simulink model "division2_repro"  (R2025b)
settings: Solver=ode4  StartTime=0.0  StopTime=40  FixedStep=dt  RelTol=1e-3
undefined symbols (not defined in the file): a0, a1, a2, a3, a4, a5, a6, a7, AgN, AgP, CNrt, CPrt, dt, EQ_intensity, EQ_sw, feedthrough_matrix_cb, feedthrough_matrix_guyan, feedthrough_matrix_original, G_1, G_2, G_3, Gss, Gss_1, KNbar_inv, KPbar_inv, KPrt, KRrt, lN, locate, locate3, lP, Mf, MNrt, MPrt, MRrt, output_matrix_cb, output_matrix_guyan, output_matrix_original, RNbar, RPbar, T, T_cb
libraries: simulink x1, sldrtlib x1
settings Model: Creator=icu327  LastModifiedBy=lenovo
settings DataIOCC: SaveFormat=Array  ReturnWorkspaceOutputs=off
settings DebuggingCC: UnconnectedInputMsg=warning  UnconnectedOutputMsg=warning  UnconnectedLineMsg=warning  ArithmeticOperatorsInVariantConditions=warning
settings HardwareCC: ProdBitPerLong=64.0  ProdHWDeviceType=Intel->x86-64 (Linux 64)
settings ModelReferenceCC: EnableRefExpFcnMdlSchedulingChecks=on
settings SFSimCC: CustomCodeUndefinedFunction=UseInterfaceOnly
settings RTWCC: SystemTargetFile=sldrt.tlc  TemplateMakefile=sldrt.tmf  RTWCompilerOptimization=on  GPUComputeCapability=3.5  Description=Simulink Desktop Real-Time
settings CodeAppCC: MaxIdLength=95.0  StateflowObjectComments=on
settings SimulinkDesktopRealTimeCC: ExtModeTransport=0.0  ExtModeStaticAllocSize=1000000.0  TargetLibSuffix=_sldrt.a  TargetPreCompLibLocation=D:\Downlad\Matlab\toolbox\sldrt\lib\win64  MultiwordLength=2048.0  DynamicStringBufferSize=256.0  ParMdlRefBuildCompliant=on  PreserveMATLABNamespacesInGeneratedCode=on  SubcomponentCodeInterfacePackaging=Reusable function

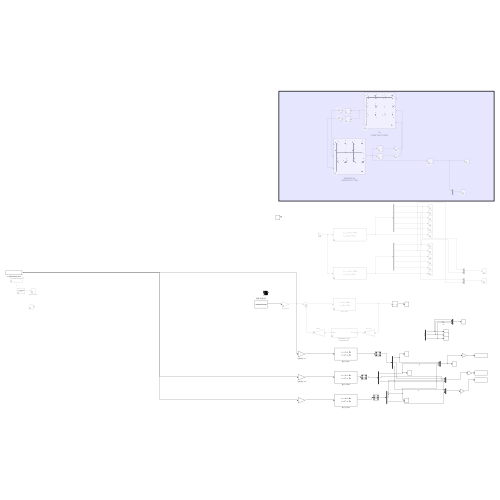
[thumbnail: Simulink's stored preview of the top-level diagram]
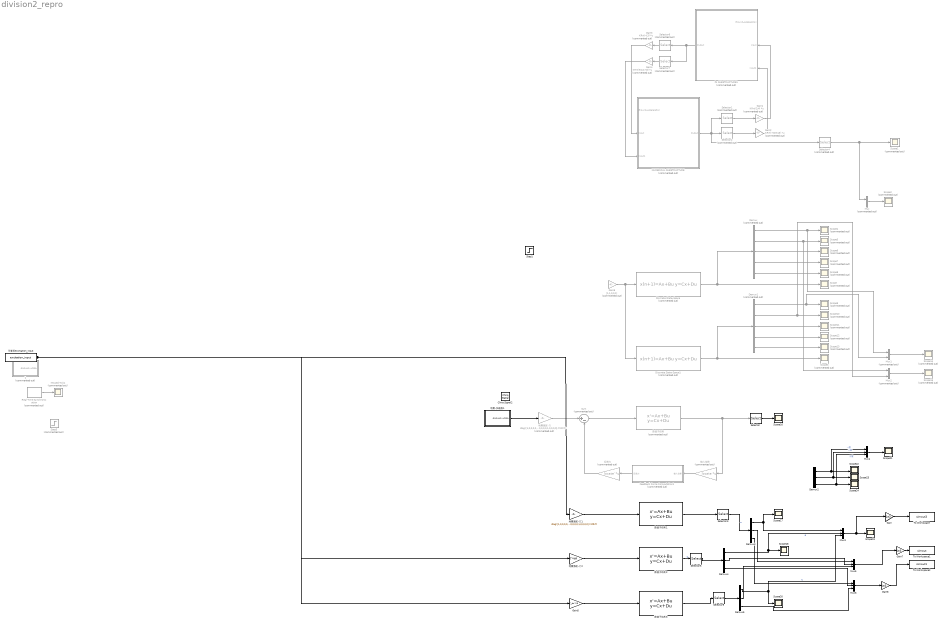
== system division2_repro ==
  " 1" : Subsystem  Commented=on
  " NUMERICAL SUBSTRUCTURE" : Subsystem  Commented=on
      mask Display: image('$imagefile'); % Use "Edit Image" on toolstrip to change.
  " Ps SUBSTRUCTURE1" : Subsystem  Commented=on
      mask Display: image('$imagefile'); % Use "Edit Image" on toolstrip to change.
  " 地震-加速度1" : Subsystem
  Chirp Signal2 : simulink/Sources/Chirp Signal  f1=0.1  T=40  f2=10
  Demux : Demux  Commented=on  Outputs=5
  Demux1 : Demux  Commented=on  Outputs=5
  Demux{2..5} (4 alike) : Demux  Outputs=3
  Discrete State-Space : DiscreteStateSpace  Commented=on  A=Gss.A  B=Gss.B  C=Gss.C  D=Gss.D  SampleTime=-1
  Discrete State-Space1 : DiscreteStateSpace  Commented=on  A=Gss_1.A  B=Gss_1.B  C=Gss_1.C  D=Gss_1.D  SampleTime=-1
  Feedback Force Computation1 : Subsystem  Commented=on
  Gain : Gain  Gain=1e3
  Gain1 : Gain  Commented=on  Gain=KRrt(3,4)  Multiplication=Matrix(K*u) (u vector)
  Gain2 : Gain  Commented=on  Gain=KRrt(7:8,9:13)  Multiplication=Matrix(K*u) (u vector)
  Gain3 : Gain  Commented=on  Gain=KRrt(4,3)  Multiplication=Matrix(K*u) (u vector)
  Gain4 : Gain  Commented=on  Gain=KRrt(9:13,7:8)  Multiplication=Matrix(K*u) (u vector)
  Gain5 : Gain  Gain=T_cb'*Mf
  Gain6 : Gain  Commented=on  Gain=[1,1,0,0,1]
  Gain7 : Gain  Gain=1e3
  Gain8 : Gain  Gain=1e3
  Missed Ticks : Scope  Commented=on
      settings: ActiveDisplayYMinimum=-21.375  ActiveDisplayYMaximum=192.375
  Mux : Mux  Commented=on  Inputs=2
  Mux1 : Mux  Commented=on  Inputs=2
  Mux2 : Mux  Commented=on  Inputs=2
  Mux{3..6} (4 alike) : Mux  Inputs=3
  Real-Time Synchronization : sldrtlib/Real-Time Synchronization  Commented=on  SampleTime=dt  MaxMissedTicks=10000  ShowMissedTicks=on  YieldWhenWaiting=off
  Scope{,1..15} (16 alike) : Scope  Commented=on
      Scope settings: ActiveDisplayYMinimum=-8E-7  ActiveDisplayYMaximum=7E-7
      Scope1 settings: ActiveDisplayYMinimum=-448565.92172  ActiveDisplayYMaximum=49840.65797
      Scope10 settings: ActiveDisplayYMinimum=-3.7E-6  ActiveDisplayYMaximum=3.7E-6
      Scope11 settings: ActiveDisplayYMinimum=-6E-6  ActiveDisplayYMaximum=6E-6  DataLoggingVariableName=ScopeData2
      Scope12 settings: ActiveDisplayYMinimum=-7E-6  ActiveDisplayYMaximum=7E-6  DataLoggingVariableName=ScopeData3
      Scope13 settings: ActiveDisplayYMinimum=-7E-7  ActiveDisplayYMaximum=7E-7  DataLoggingVariableName=ScopeData4
      Scope14 settings: ActiveDisplayYMinimum=-6E-7  ActiveDisplayYMaximum=7E-7  DataLoggingVariableName=ScopeData7
      Scope15 settings: ActiveDisplayYMinimum=-1.6E-6  ActiveDisplayYMaximum=1.7E-6
      Scope2 settings: ActiveDisplayYMinimum=-448565.92172  ActiveDisplayYMaximum=49840.65797  DataLoggingVariableName=ScopeData2
      Scope3 settings: ActiveDisplayYMinimum=-2.5E-6  ActiveDisplayYMaximum=2.5E-6  DataLoggingVariableName=ScopeData5
      Scope4 settings: ActiveDisplayYMinimum=-2.5E-8  ActiveDisplayYMaximum=3.7E-8  DataLoggingVariableName=ScopeData3
      Scope5 settings: ActiveDisplayYMinimum=-3.7E-6  ActiveDisplayYMaximum=3.7E-6  DataLoggingVariableName=ScopeData4
      Scope6 settings: ActiveDisplayYMinimum=-6E-6  ActiveDisplayYMaximum=6E-6  DataLoggingVariableName=ScopeData5
      Scope7 settings: ActiveDisplayYMinimum=-7E-6  ActiveDisplayYMaximum=7E-6  DataLoggingVariableName=ScopeData6
      Scope8 settings: ActiveDisplayYMinimum=-7E-7  ActiveDisplayYMaximum=7E-7  DataLoggingVariableName=ScopeData7
      Scope9 settings: ActiveDisplayYMinimum=-2.5E-8  ActiveDisplayYMaximum=3.7E-8  DataLoggingVariableName=ScopeData6
  Scope{16..24} (9 alike) : Scope
      Scope16 settings: ActiveDisplayYMinimum=-4.1813024288037124E+278  ActiveDisplayYMaximum=3.7631721859233419E+279
      Scope17 settings: ActiveDisplayYMinimum=-0.00351  ActiveDisplayYMaximum=0.00404
      Scope18 settings: ActiveDisplayYMinimum=-0.00375  ActiveDisplayYMaximum=0.00378  DataLoggingVariableName=ScopeData2
      Scope19 settings: ActiveDisplayYMinimum=-0.01112  ActiveDisplayYMaximum=0.00785  DataLoggingVariableName=ScopeData3
      Scope20 settings: ActiveDisplayYMinimum=-0.00351  ActiveDisplayYMaximum=0.00404  DataLoggingVariableName=ScopeData4
      Scope21 settings: ActiveDisplayYMinimum=-0.01512  ActiveDisplayYMaximum=0.0154
      Scope22 settings: ActiveDisplayYMinimum=-0.00351  ActiveDisplayYMaximum=0.00405  DataLoggingVariableName=ScopeData2
      Scope23 settings: ActiveDisplayYMinimum=-0.00973  ActiveDisplayYMaximum=0.01044  DataLoggingVariableName=ScopeData3
      Scope24 settings: ActiveDisplayYMinimum=-0.01512  ActiveDisplayYMaximum=0.0154  DataLoggingVariableName=ScopeData4
  Selector : Selector  InputPortWidth=15  IndexOptions=Index vector (dialog)  Indices=[1]  OutputSizes=1
  Selector1 : Selector  Commented=on  InputPortWidth=11  IndexOptions=Index vector (dialog)  Indices=[2]  OutputSizes=1
  Selector2 : Selector  Commented=on  InputPortWidth=11  IndexOptions=Index vector (dialog)  Indices=[5 6 7 8 9]  OutputSizes=1
  Selector3 : Selector  InputPortWidth=3  IndexOptions=Index vector (dialog)  Indices=[1 2 3]  OutputSizes=1
  Selector4 : Selector  Commented=on  InputPortWidth=11  IndexOptions=Index vector (dialog)  Indices=[1]  OutputSizes=1
  Selector5 : Selector  InputPortWidth=3  IndexOptions=Index vector (dialog)  Indices=[1 2 3]  OutputSizes=1
  Selector6 : Selector  Commented=on  InputPortWidth=6  IndexOptions=Index vector (dialog)  Indices=[3]  OutputSizes=1
  Selector7 : Selector  Commented=on  InputPortWidth=6  IndexOptions=Index vector (dialog)  Indices=[5 6]  OutputSizes=1
  Selector9 : Selector  InputPortWidth=3  IndexOptions=Index vector (dialog)  Indices=[1 2 3]  OutputSizes=1
  Step1 : Step  SampleTime=0
  Step5 : Step  Commented=on  SampleTime=0
  Sum : Sum  Commented=on  Inputs=|+-
  To Workspace : ToWorkspace  VariableName=simout3  SaveFormat=Timeseries  SampleTime=-1
  To Workspace1 : ToWorkspace  VariableName=simout  SaveFormat=Timeseries  SampleTime=-1
  To Workspace2 : ToWorkspace  VariableName=simout1  SaveFormat=Timeseries  SampleTime=-1
  反馈力 : Gain  Commented=on  Gain=locate'  Multiplication=Matrix(K*u) (u vector)
  可复现excitation_input : FromWorkspace  VariableName=excitation_input  OutputAfterFinalValue=Holding final value
  地震激励-力 : Gain  Commented=on  Gain=diag([1,0,0,0,0,1,0,0,0,0,1,0,0,0,0].*MRrt)
  地震激励-力1 : Gain  Gain=diag([1,0,0,0,0,1,0,0,0,0,1,0,0,0,0].*MRrt)
  地震激励-力2 : Gain  Gain=T'*Mf
  数值子结构 : StateSpace  Commented=on  InitialCondition=0
  数值子结构1 : StateSpace  A=G_1.A  B=G_1.B  C=output_matrix_original  D=feedthrough_matrix_original  InitialCondition=0
  数值子结构2 : StateSpace  A=G_2.A  B=G_2.B  C=output_matrix_guyan  D=feedthrough_matrix_guyan  InitialCondition=0
  数值子结构3 : StateSpace  A=G_3.A  B=G_3.B  C=output_matrix_cb  D=feedthrough_matrix_cb  InitialCondition=0
  输入位移 : Gain  Commented=on  Gain=locate  Multiplication=Matrix(K*u) (u vector)
  wires:
  Real-Time Synchronization/1 -> Missed Ticks/1
  Mux/1 -> Scope2/1
  " Ps SUBSTRUCTURE1"/1(Output) -> Selector7/1, Selector6/1
  Selector4/1 -> Scope1/1, Mux/1
  Selector2/1 -> Gain2/1
  Selector1/1 -> Gain1/1
  Gain1/1 -> " Ps SUBSTRUCTURE1"/2(Input)
  Gain2/1 -> " Ps SUBSTRUCTURE1"/3(Input1)
  Selector6/1 -> Gain3/1
  Gain3/1 -> " NUMERICAL SUBSTRUCTURE"/2(Input)
  Selector7/1 -> Gain4/1
  Gain4/1 -> " NUMERICAL SUBSTRUCTURE"/3(Input1)
  " NUMERICAL SUBSTRUCTURE"/1(Output) -> Selector4/1, Selector1/1, Selector2/1
  Discrete State-Space/1 -> Demux/1, Scope/1
  Demux/1 -> Mux1/1, Scope4/1
  Demux/2 -> Mux2/1, Scope5/1
  Demux/4 -> Scope7/1
  Demux/5 -> Scope8/1
  Demux1/5 -> Scope13/1
  Demux1/4 -> Scope12/1
  Demux1/1 -> Mux1/2, Scope9/1
  Discrete State-Space1/1 -> Demux1/1, Scope3/1
  Gain6/1 -> Discrete State-Space1/1, Discrete State-Space/1
  Demux1/3 -> Scope11/1
  Mux1/1 -> Scope14/1
  Mux2/1 -> Scope15/1
  Demux1/2 -> Mux2/2, Scope10/1
  Demux/3 -> Scope6/1
  Selector/1 -> Scope16/1
  数值子结构/1 -> 输入位移/1, Selector/1
  Feedback Force Computation1/1(反馈力) -> 反馈力/1
  输入位移/1 -> Feedback Force Computation1/1(输入位移)
  地震激励-力/1 -> Sum/1
  Sum/1 -> 数值子结构/1
  反馈力/1 -> Sum/2
  数值子结构1/1 -> Selector3/1
  地震激励-力1/1 -> 数值子结构1/1
  地震激励-力2/1 -> 数值子结构2/1
  Demux4/1 -> Scope18/1, Mux3/2  "g"
  Mux3/1 -> Gain/1, Scope19/1
  " 地震-加速度1"/1(GROUND ACCEL) -> 地震激励-力/1
  数值子结构3/1 -> Selector9/1
  Demux5/1 -> Mux3/3, Scope20/1  "C"
  Gain5/1 -> 数值子结构3/1
  Demux2/1 -> Mux4/1, Scope22/1  "一层"
  Demux2/2 -> Mux4/2, Scope23/1  "二层"
  Demux2/3 -> Mux4/3, Scope24/1  "三层"
  Mux4/1 -> Scope21/1
  Selector3/1 -> Demux3/1  "o"
  Demux3/1 -> Mux3/1, Scope17/1
  数值子结构2/1 -> Selector5/1  "g"
  Selector9/1 -> Demux5/1
  Demux3/2 -> Mux5/1
  Demux4/2 -> Mux5/2
  Demux5/2 -> Mux5/3
  Demux3/3 -> Mux6/1
  Mux5/1 -> Gain7/1
  Mux6/1 -> Gain8/1
  Gain/1 -> To Workspace/1
  Gain7/1 -> To Workspace1/1
  Gain8/1 -> To Workspace2/1
  Selector5/1 -> Demux4/1
  可复现excitation_input/1 -> 地震激励-力1/1, 地震激励-力2/1, Gain5/1
  Demux4/3 -> Mux6/2
  Demux5/3 -> Mux6/3

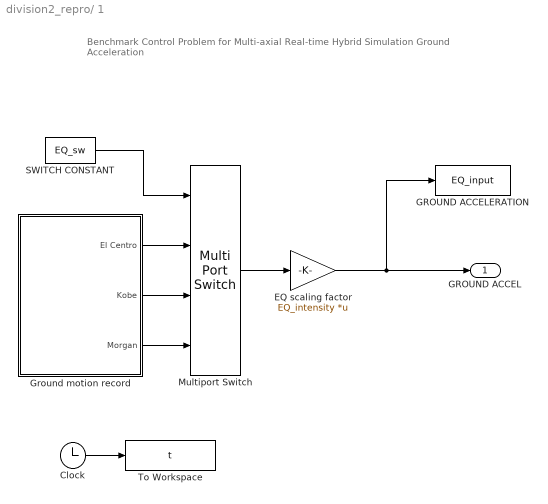
== system division2_repro/ 1 ==
  note: Benchmark Control Problem for
      | Multi-axial Real-time Hybrid Simulation
      | Ground Acceleration
  Clock : Clock
  EQ scaling factor : Gain  Gain=EQ_intensity  Multiplication=Matrix(K*u)
  GROUND ACCELERATION : ToWorkspace  VariableName=EQ_input  SampleTime=-1
      settings: Save2DSignal=2-D array (concatenate along first dimension)
  Ground motion record : Subsystem
  Multiport Switch : MultiPortSwitch  SaturateOnIntegerOverflow=off  InputSameDT=off
  SWITCH CONSTANT : Constant  Value=EQ_sw
  To Workspace : ToWorkspace  VariableName=t  SampleTime=dt
  GROUND ACCEL : Outport  VectorParamsAs1DForOutWhenUnconnected=off
  wires:
  Multiport Switch/1 -> EQ scaling factor/1
  EQ scaling factor/1 -> GROUND ACCELERATION/1, GROUND ACCEL/1
  Ground motion record/1(El Centro) -> Multiport Switch/2
  Ground motion record/2(Kobe) -> Multiport Switch/3
  Ground motion record/3(Morgan) -> Multiport Switch/4
  SWITCH CONSTANT/1 -> Multiport Switch/1
  Clock/1 -> To Workspace/1

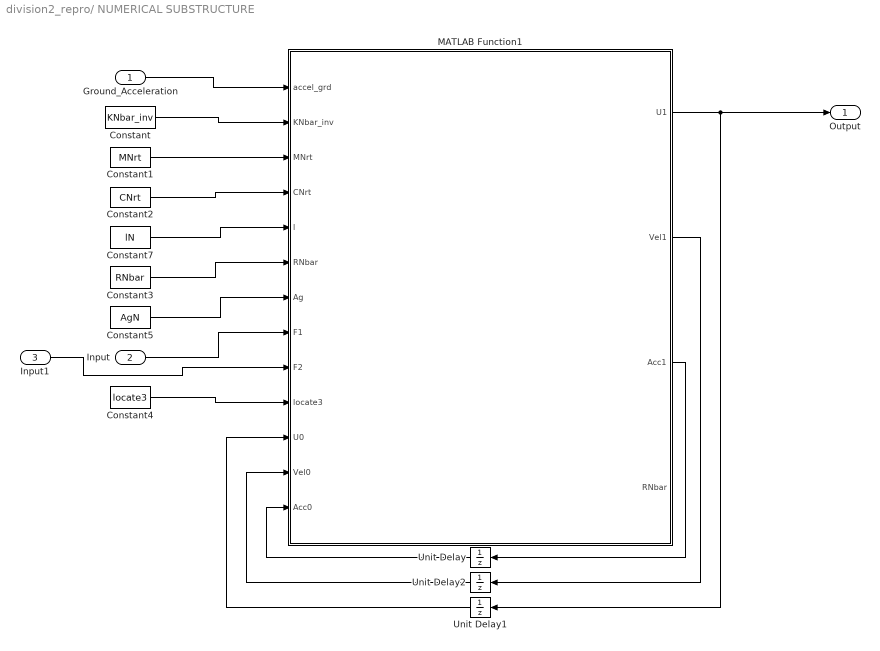
== system division2_repro/ NUMERICAL SUBSTRUCTURE ==
  Ground_Acceleration : Inport
  Input : Inport  Port=2
  Input1 : Inport  Port=3
  Constant : Constant  Value=KNbar_inv  VectorParams1D=off
  Constant1 : Constant  Value=MNrt  VectorParams1D=off
  Constant2 : Constant  Value=CNrt  VectorParams1D=off
  Constant3 : Constant  Value=RNbar  VectorParams1D=off
  Constant4 : Constant  Value=locate3  VectorParams1D=off
  Constant5 : Constant  Value=AgN  VectorParams1D=off
  Constant7 : Constant  Value=lN  VectorParams1D=off
  MATLAB Function1 : MATLAB Function  TreatAsAtomicUnit=on
  Unit Delay : UnitDelay  SampleTime=-1  HasFrameUpgradeWarning=on
  Unit Delay1 : UnitDelay  SampleTime=-1  HasFrameUpgradeWarning=on
  Unit Delay2 : UnitDelay  SampleTime=-1  HasFrameUpgradeWarning=on
  Output : Outport
  wires:
  Ground_Acceleration/1 -> MATLAB Function1/1(accel_grd)
  Constant/1 -> MATLAB Function1/2(KNbar_inv)
  Constant1/1 -> MATLAB Function1/3(MNrt)
  Constant2/1 -> MATLAB Function1/4(CNrt)
  Constant7/1 -> MATLAB Function1/5(l)
  Unit Delay2/1 -> MATLAB Function1/12(Vel0)
  Unit Delay/1 -> MATLAB Function1/13(Acc0)
  MATLAB Function1/2(Vel1) -> Unit Delay2/1
  MATLAB Function1/3(Acc1) -> Unit Delay/1
  Constant5/1 -> MATLAB Function1/7(Ag)
  Unit Delay1/1 -> MATLAB Function1/11(U0)
  Constant3/1 -> MATLAB Function1/6("RNbar ")
  Input/1 -> MATLAB Function1/8(F1)
  MATLAB Function1/1(U1) -> Output/1, Unit Delay1/1
  Constant4/1 -> MATLAB Function1/10(locate3)
  Input1/1 -> MATLAB Function1/9(F2)

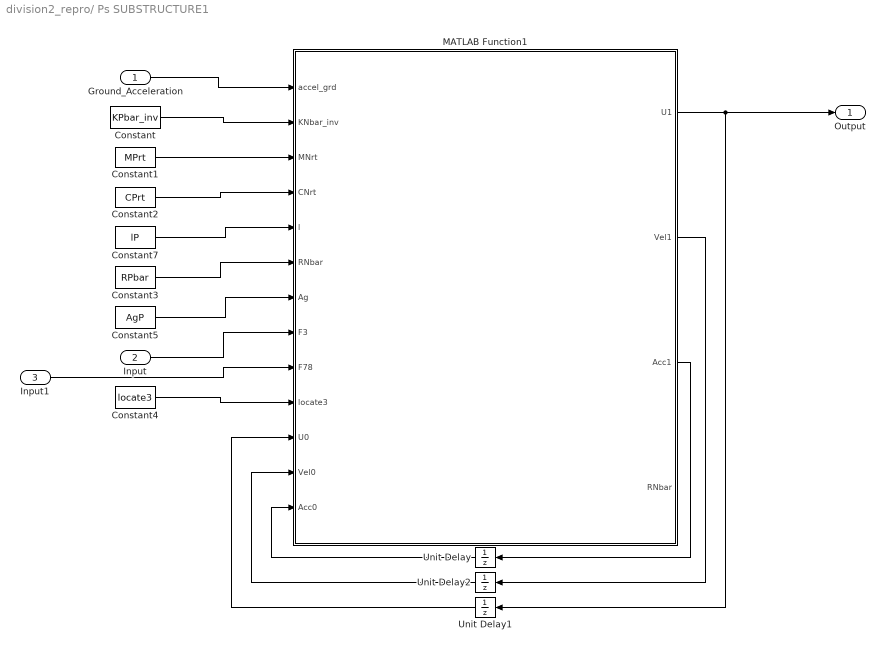
== system division2_repro/ Ps SUBSTRUCTURE1 ==
  Ground_Acceleration : Inport
  Input : Inport  Port=2
  Input1 : Inport  Port=3
  Constant : Constant  Value=KPbar_inv  VectorParams1D=off
  Constant1 : Constant  Value=MPrt  VectorParams1D=off
  Constant2 : Constant  Value=CPrt  VectorParams1D=off
  Constant3 : Constant  Value=RPbar  VectorParams1D=off
  Constant4 : Constant  Value=locate3  VectorParams1D=off
  Constant5 : Constant  Value=AgP  VectorParams1D=off
  Constant7 : Constant  Value=lP  VectorParams1D=off
  MATLAB Function1 : MATLAB Function  TreatAsAtomicUnit=on
  Unit Delay : UnitDelay  SampleTime=-1  HasFrameUpgradeWarning=on
  Unit Delay1 : UnitDelay  SampleTime=-1  HasFrameUpgradeWarning=on
  Unit Delay2 : UnitDelay  SampleTime=-1  HasFrameUpgradeWarning=on
  Output : Outport
  wires:
  Ground_Acceleration/1 -> MATLAB Function1/1(accel_grd)
  Constant/1 -> MATLAB Function1/2(KNbar_inv)
  Constant1/1 -> MATLAB Function1/3(MNrt)
  Constant2/1 -> MATLAB Function1/4(CNrt)
  Constant7/1 -> MATLAB Function1/5(l)
  Unit Delay2/1 -> MATLAB Function1/12(Vel0)
  Unit Delay/1 -> MATLAB Function1/13(Acc0)
  MATLAB Function1/2(Vel1) -> Unit Delay2/1
  MATLAB Function1/3(Acc1) -> Unit Delay/1
  Constant5/1 -> MATLAB Function1/7(Ag)
  Unit Delay1/1 -> MATLAB Function1/11(U0)
  Constant3/1 -> MATLAB Function1/6("RNbar ")
  Input/1 -> MATLAB Function1/8(F3)
  MATLAB Function1/1(U1) -> Output/1, Unit Delay1/1
  Constant4/1 -> MATLAB Function1/10(locate3)
  Input1/1 -> MATLAB Function1/9(F78)

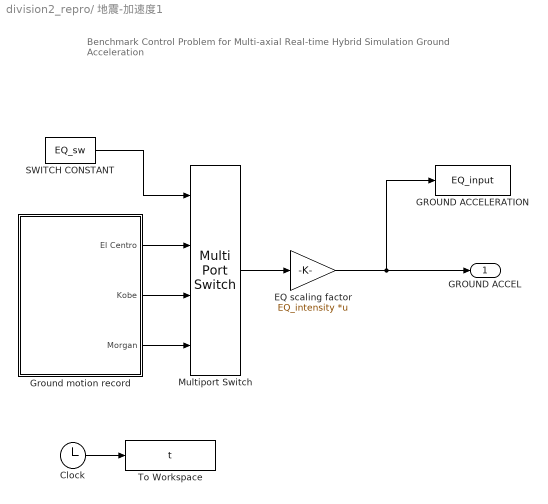
== system division2_repro/ 地震-加速度1 ==
  note: Benchmark Control Problem for
      | Multi-axial Real-time Hybrid Simulation
      | Ground Acceleration
  Clock : Clock
  EQ scaling factor : Gain  Gain=EQ_intensity  Multiplication=Matrix(K*u)
  GROUND ACCELERATION : ToWorkspace  VariableName=EQ_input  SampleTime=-1
      settings: Save2DSignal=2-D array (concatenate along first dimension)
  Ground motion record : Subsystem
  Multiport Switch : MultiPortSwitch  SaturateOnIntegerOverflow=off  InputSameDT=off
  SWITCH CONSTANT : Constant  Value=EQ_sw
  To Workspace : ToWorkspace  VariableName=t  SampleTime=dt
  GROUND ACCEL : Outport  VectorParamsAs1DForOutWhenUnconnected=off
  wires:
  Multiport Switch/1 -> EQ scaling factor/1
  EQ scaling factor/1 -> GROUND ACCELERATION/1, GROUND ACCEL/1
  Ground motion record/1(El Centro) -> Multiport Switch/2
  Ground motion record/2(Kobe) -> Multiport Switch/3
  Ground motion record/3(Morgan) -> Multiport Switch/4
  SWITCH CONSTANT/1 -> Multiport Switch/1
  Clock/1 -> To Workspace/1

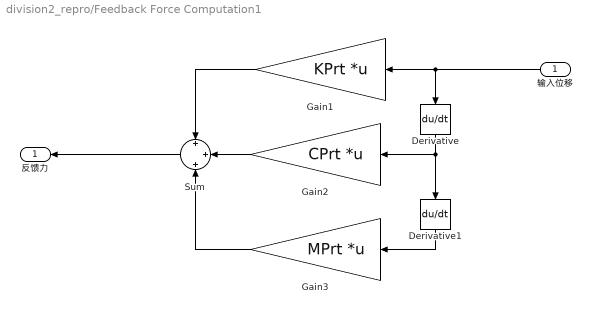
== system division2_repro/Feedback Force Computation1 ==
  输入位移 : Inport
  Derivative : Derivative
  Derivative1 : Derivative
  Gain1 : Gain  Gain=KPrt  Multiplication=Matrix(K*u) (u vector)
  Gain2 : Gain  Gain=CPrt  Multiplication=Matrix(K*u) (u vector)
  Gain3 : Gain  Gain=MPrt  Multiplication=Matrix(K*u) (u vector)
  Sum : Sum  Inputs=+|+|+
  反馈力 : Outport
  wires:
  Gain2/1 -> Sum/2
  Derivative/1 -> Derivative1/1, Gain2/1
  Gain1/1 -> Sum/1
  Sum/1 -> 反馈力/1
  输入位移/1 -> Derivative/1, Gain1/1
  Derivative1/1 -> Gain3/1
  Gain3/1 -> Sum/3

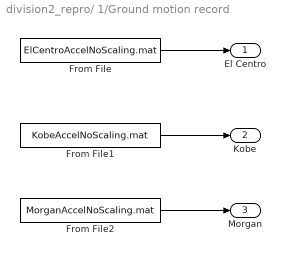
== system division2_repro/ 1/Ground motion record ==
  From File : FromFile  FileName=ElCentroAccelNoScaling.mat  SampleTime=dt
  From File1 : FromFile  FileName=KobeAccelNoScaling.mat  SampleTime=dt
  From File2 : FromFile  FileName=MorganAccelNoScaling.mat  SampleTime=dt
  El Centro : Outport
  Kobe : Outport  Port=2
  Morgan : Outport  Port=3
  wires:
  From File/1 -> El Centro/1
  From File2/1 -> Morgan/1
  From File1/1 -> Kobe/1

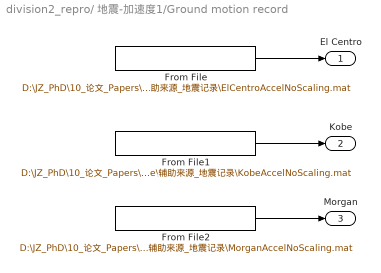
== system division2_repro/ 地震-加速度1/Ground motion record ==
  From File : FromFile  FileName=D:\JZ_PhD\10_论文_Papers\Li\RHTS\liangyustability-master\test\00_失败尝试与候选路线\板块18_图3-5至图3-15逐图计算复现\input\author_source\辅助来源_地震记录\ElCentroAccelNoScaling.mat  SampleTime=dt
  From File1 : FromFile  FileName=D:\JZ_PhD\10_论文_Papers\Li\RHTS\liangyustability-master\test\00_失败尝试与候选路线\板块18_图3-5至图3-15逐图计算复现\input\author_source\辅助来源_地震记录\KobeAccelNoScaling.mat  SampleTime=dt
  From File2 : FromFile  FileName=D:\JZ_PhD\10_论文_Papers\Li\RHTS\liangyustability-master\test\00_失败尝试与候选路线\板块18_图3-5至图3-15逐图计算复现\input\author_source\辅助来源_地震记录\MorganAccelNoScaling.mat  SampleTime=dt
  El Centro : Outport
  Kobe : Outport  Port=2
  Morgan : Outport  Port=3
  wires:
  From File/1 -> El Centro/1
  From File2/1 -> Morgan/1
  From File1/1 -> Kobe/1

== matlab function division2_repro/ Ps SUBSTRUCTURE1/MATLAB Function1 ==
  data: U1 output; Vel1 output; Acc1 output; accel_grd input; KNbar_inv input; MNrt input; CNrt input; l input; RNbar input; Ag input; F3 input; F78 input; locate3 input; U0 input; Vel0 input; Acc0 input; a0 parameter; a1 parameter; a2 parameter; a3 parameter; a4 parameter; a5 parameter; a6 parameter; a7 parameter; RNbar output
function [U1,Vel1,Acc1,RNbar]=fcn2(accel_grd,KNbar_inv, MNrt, CNrt,l,RNbar,Ag,F3,F78,locate3,...
    U0,Vel0,Acc0, a0, a1, a2, a3, a4, a5, a6, a7)
             
    % 该求解方法为 Newmark-β法        
    % ============================
	% *  Update next iteration   *
	% ============================
    ndof = length(KNbar_inv);
    U1   = zeros(ndof,1);
    Vel1 = zeros(ndof,1);
    Acc1 = zeros(ndof,1);
    F = zeros(6,1);
    F(3,1) = F3;
    F(5:6,1) = F78;
    % ============================
	% *  Feedback Force / Moment *
	% ============================
%     F(27) = -FB_force;
%     F(14) = -FB_moment;

    % ==========================
	% *     Update Matrices    *
	% ==========================
    Ag  = accel_grd * l;
   	% ==========================
	% * 	  Form Rbar  	   *
	% ==========================
	RNbar = ( (MNrt * ((a0*U0)+(a2*Vel0)+(a3*Acc0))) + ...
		     (CNrt * ((a1*U0)+(a4*Vel0)+(a5*Acc0))) -F-  (MNrt * Ag) );
    % ==========================
	% * Solve for Displacement *
	% ==========================
	U1 = KNbar_inv * RNbar;
    
	% ============================
	% * Compute Velocity & Accel *
	% ============================
	Acc1=a0*(U1-U0)-a2*Vel0-a3*Acc0;
	Vel1=Vel0+a7*Acc1+a6*Acc0;

end

== matlab function division2_repro/ NUMERICAL SUBSTRUCTURE/MATLAB Function1 ==
  data: U1 output; Vel1 output; Acc1 output; accel_grd input; KNbar_inv input; MNrt input; CNrt input; l input; RNbar input; Ag input; F1 input; F2 input; locate3 input; U0 input; Vel0 input; Acc0 input; a0 parameter; a1 parameter; a2 parameter; a3 parameter; a4 parameter; a5 parameter; a6 parameter; a7 parameter; RNbar output
function [U1,Vel1,Acc1,RNbar]=fcn2(accel_grd,KNbar_inv, MNrt, CNrt,l,RNbar,Ag,F1,F2,locate3,...
    U0,Vel0,Acc0, a0, a1, a2, a3, a4, a5, a6, a7)
             
    % 该求解方法为 Newmark-β法        
    % ============================
	% *  Update next iteration   *
	% ============================
    ndof = length(KNbar_inv);
    U1   = zeros(ndof,1);
    Vel1 = zeros(ndof,1);
    Acc1 = zeros(ndof,1);
    F = zeros(11,1);
    F(2,1) = F1;
    F(5:9) = F2;
    % ============================
	% *  Feedback Force / Moment *
	% ============================
%     F(27) = -FB_force;
%     F(14) = -FB_moment;

    % ==========================
	% *     Update Matrices    *
	% ==========================
    Ag  = accel_grd * l;
   	% ==========================
	% * 	  Form Rbar  	   *
	% ==========================
	RNbar = ( (MNrt * ((a0*U0)+(a2*Vel0)+(a3*Acc0))) + ...
		     (CNrt * ((a1*U0)+(a4*Vel0)+(a5*Acc0))) -F-  (MNrt * Ag) );
    % ==========================
	% * Solve for Displacement *
	% ==========================
	U1 = KNbar_inv * RNbar;
    
	% ============================
	% * Compute Velocity & Accel *
	% ============================
	Acc1=a0*(U1-U0)-a2*Vel0-a3*Acc0;
	Vel1=Vel0+a7*Acc1+a6*Acc0;

end
